simulink model "pq_onda"  (R2022b)
settings: Solver=ode45  StartTime=0.0  StopTime=1.5  MaxStep=1.5/57  MinStep=0.02459  RelTol=1e-3
settings Model: Creator=FELIPE OCAMPO  LastModifiedBy=Catalina

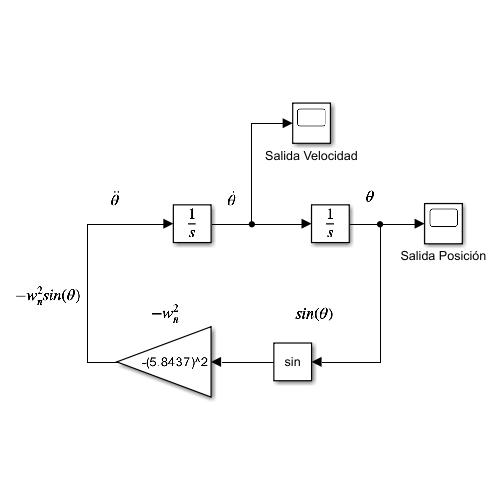
[thumbnail: Simulink's stored preview of the top-level diagram]
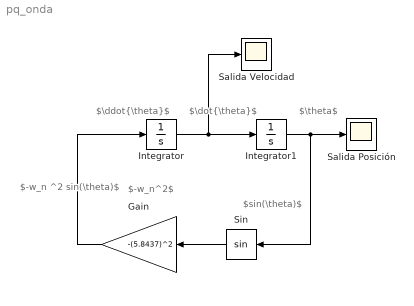
== system pq_onda ==
  note: $\dot{\theta}$
  note: $-w_n ^2 sin(\theta)$
  note: $-w_n^2$
  note: $\theta$
  note: $\ddot{\theta}$
  note: $sin(\theta)$
  Gain : Gain  Gain=-(5.8437)^2
  Integrator : Integrator
  Integrator1 : Integrator  InitialCondition=0.2531
  Salida Posición : Scope
  Salida Velocidad : Scope
  Sin : Trigonometry
  wires:
  Integrator1/1 -> Salida Posición/1, Sin/1
  Sin/1 -> Gain/1
  Gain/1 -> Integrator/1
  Integrator/1 -> Salida Velocidad/1, Integrator1/1
